simulink model "model"  (Simulink 9.2)
settings: Solver=VariableStepAuto  StartTime=0.0  StopTime=2  RelTol=1e-3
values from neighbouring files (symbols this model uses):
  beta = 25*10^4    (= 250000)    [constant.m]
  dp = 10*10^-6    (= 1e-05)    [constant.m]
  rhop = 3263    [constant.m]
  theta1 = 2.05    [constant.m]
  theta2 = 3.031    [constant.m]
  vf = 1*10^-3    (= 0.001)    [constant.m]
  x0 = 290*10^-6    (= 0.00029)    [constant.m]
  xn = 0    [constant.m]
  y0 = 25*10^-6    (= 2.5e-05)    [constant.m]
  yn = 0    [constant.m]
settings Model: Creator=lianq  LastModifiedBy=yizhan
settings DataIOCC: LimitDataPoints=off  SaveFormat=Dataset  SignalLoggingSaveFormat=Dataset
settings OptimizationCC: LifeSpan=auto
settings DebuggingCC: UnderspecifiedInitializationDetection=Simplified  MergeDetectMultiDrivingBlocksExec=error  FcnCallInpInsideContextMsg=error  StateNameClashWarn=none  SFUnexpectedBacktrackingDiag=error  SFNoUnconditionalDefaultTransitionDiag=error  SFExecutionAtInitializationDiag=warning
settings HardwareCC: ProdBitPerPointer=64  ProdBitPerSizeT=64  ProdBitPerPtrDiffT=64  ProdLargestAtomicFloat=Float  ProdIntDivRoundTo=Zero  ProdEndianess=LittleEndian  ProdWordSize=64  ProdHWDeviceType=Intel->x86-64 (Windows64)
settings ModelReferenceCC: PropagateSignalLabelsOutOfModel=on
settings SFSimCC: SimUseLocalCustomCode=on
settings RTWCC: RTWUseLocalCustomCode=on
settings CodeAppCC: StateflowObjectComments=off
settings GRTTargetCC: TargetLangStandard=C99 (ISO)  GeneratePreprocessorConditionals=Use local settings  CombineOutputUpdateFcns=on  GRTInterface=off
settings ConfigComp: CovMetricSettings=dwe  CovHtmlReporting=off  CovSaveCumulativeToWorkspaceVar=off  CovSaveSingleToWorkspaceVar=off  CovExternalEMLEnable=on

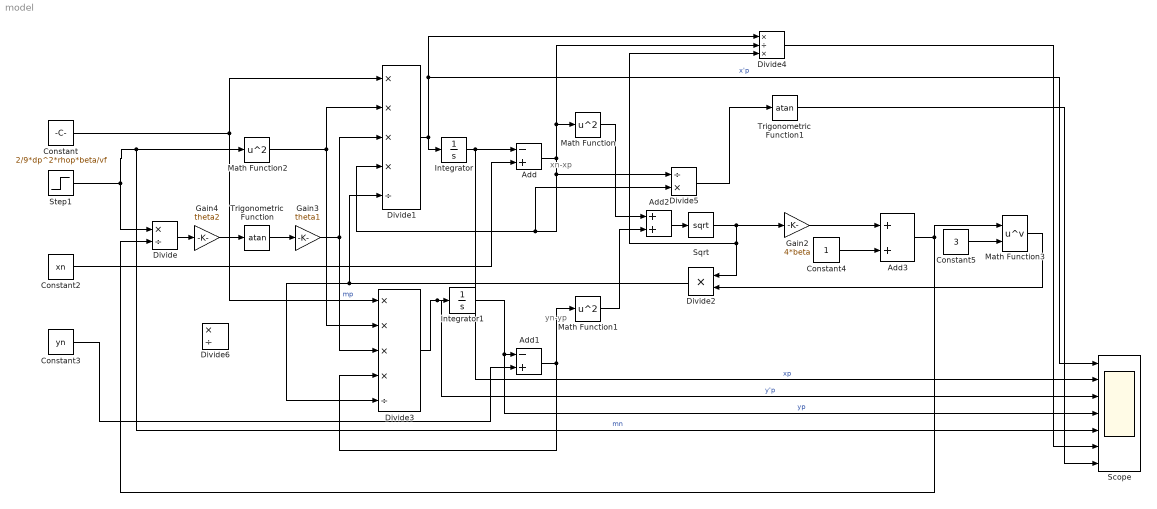
== system model ==
  note: yn-yp
  note: xn-xp
  Add : Sum  Inputs=-+
  Add1 : Sum  Inputs=-+
  Add2 : Sum
  Add3 : Sum
  Constant : Constant  Value=2/9*dp^2*rhop*beta/vf
  Constant2 : Constant  Value=xn
  Constant3 : Constant  Value=yn
  Constant4 : Constant
  Constant5 : Constant  Value=3
  Divide : Product  Inputs=*/
  Divide1 : Product  Inputs=****/
  Divide2 : Product  Inputs=**
  Divide3 : Product  Inputs=****/
  Divide4 : Product  Inputs=*/*
  Divide5 : Product  Inputs=/*
  Divide6 : Product  Inputs=*/
  Gain2 : Gain  Gain=4*beta
  Gain3 : Gain  Gain=theta1
  Gain4 : Gain  Gain=theta2
  Integrator : Integrator  InitialCondition=x0
  Integrator1 : Integrator  InitialCondition=y0
  Math Function : Math  Operator=square  SaturateOnIntegerOverflow=on
  Math Function1 : Math  Operator=square  SaturateOnIntegerOverflow=on
  Math Function2 : Math  Operator=square  SaturateOnIntegerOverflow=on
  Math Function3 : Math  Operator=pow  SaturateOnIntegerOverflow=on
  Scope : Scope  NumInputPorts=7
  Sqrt : Sqrt  SaturateOnIntegerOverflow=on
  Step1 : Step  Time=0  After=10  SampleTime=0
  Trigonometric Function : Trigonometry  Operator=atan
  Trigonometric Function1 : Trigonometry  Operator=atan
  wires:
  Divide1/1 -> Integrator/1, Divide4/1, Scope/1  "x'p"
  Constant/1 -> Divide3/1, Divide1/1
  Divide3/1 -> Scope/3, Integrator1/1  "y'p"
  Integrator/1 -> Scope/2, Add/1  "xp"
  Constant2/1 -> Add/2
  Constant3/1 -> Add1/2
  Integrator1/1 -> Scope/4, Add1/1  "yp"
  Add/1 -> Divide4/2, Math Function/1, Divide5/1, Divide5/2, Divide1/4
  Add1/1 -> Math Function1/1, Divide3/4
  Math Function/1 -> Add2/1
  Math Function1/1 -> Add2/2
  Add2/1 -> Sqrt/1
  Sqrt/1 -> Divide4/3, Divide2/1, Gain2/1
  Gain2/1 -> Add3/1
  Constant4/1 -> Add3/2
  Add3/1 -> Divide/2, Math Function3/1
  Step1/1 -> Scope/5, Math Function2/1, Divide/1  "mn"
  Divide/1 -> Gain4/1
  Gain4/1 -> Trigonometric Function/1
  Trigonometric Function/1 -> Gain3/1
  Gain3/1 -> Divide1/3, Divide3/3  "mp"
  Math Function2/1 -> Divide3/2, Divide1/2
  Constant5/1 -> Math Function3/2
  Math Function3/1 -> Divide2/2
  Divide2/1 -> Divide1/5, Divide3/5
  Divide4/1 -> Scope/6
  Divide5/1 -> Trigonometric Function1/1
  Trigonometric Function1/1 -> Scope/7
